simulink library "takeOffToLandingExp"  (R2020a)
settings: Solver=VariableStepAuto  StartTime=0.0  StopTime=10.0  RelTol=1e-3
undefined symbols (not defined in the file or in its folder): elSP, env, FLIGHTCONTROLLER, fltCtrl, gain2to3, gain4to1, hiLvlCtrl, initializeBussesFromBlock, pathFollowingControllerExp, pathFollowingControllerExp_cl, vhcl
libraries: simulink x9, filteredPIDController_ul x4, ctrlAllocMatrix_cl x3, velocityAngle_ul x3, hiToLoElevationControllerExp x2, takeoffToLanding_cl x2, dspsigops x1, setpointToOutput_cl x1, stopwatch_ul x1, courseFollowExp_cl x1, eulAng2RotMat_ul x1, angleBtw2Vecs_ul x1
settings Model: Creator=jcreed2  LastModifiedBy=jcreed2

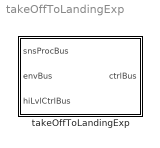
== system takeOffToLandingExp ==
  takeOffToLandingExp : Subsystem  LoadFcn=initializeBussesFromBlock(gcb)  InitFcn=initializeBussesFromBlock(gcb)  StartFcn=initializeBussesFromBlock(gcb)  mask{initPosForInitSStar=vhcl.initPosVecGnd.Value, fluidDensity=env.water.density.Value, pathCtrl=fltCtrl, aeroStruct=vhcl.struct('OCT.aeroSurf')}
      mask prompts: initPosForInitSStar "Initial Position"; fluidDensity "Fluid Density"; pathCtrl "Controller"; aeroStruct "Aerodynamic Structure"

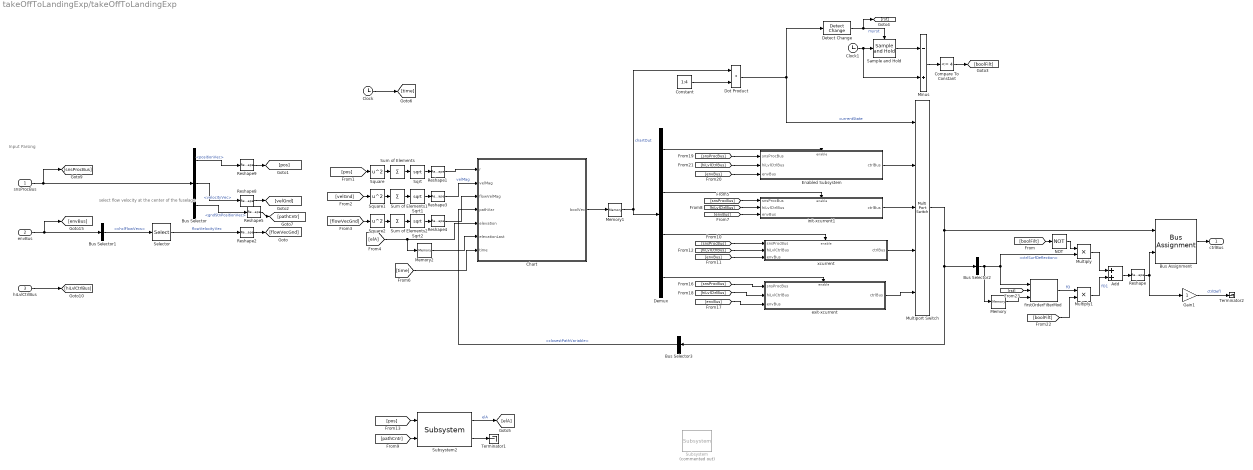
== system takeOffToLandingExp/takeOffToLandingExp ==
  note: select flow velocity at the center of the fuselage
  note: Input Parsing
  snsProcBus : Inport  OutDataTypeStr=Bus: sensorsProcessingBus
  envBus : Inport  Port=2  OutDataTypeStr=Bus: envBus
  hiLvlCtrlBus : Inport  Port=3  OutDataTypeStr=Bus: hiLvlCtrlBus
  Add : Sum
  Bus Assignment : BusAssignment  AssignedSignals=ctrlSurfDeflection
  Bus Selector : BusSelector  OutputSignals=positionVec,velocityVec,gndStnPositionVec
  Bus Selector1 : BusSelector  OutputSignals=vhclFlowVecs
  Bus Selector2 : BusSelector  OutputSignals=ctrlSurfDeflection
  Bus Selector3 : BusSelector  OutputSignals=closestPathVariable
  Chart : Stateflow chart  AncestorBlock=takeoffToLanding_cl/takeoffToLanding/Chart  TreatAsAtomicUnit=on  mask{nonCrossSpoolGain=2, gain41=gain4to1, gain23=gain2to3, maxR=3}
      mask prompts: nonCrossSpoolGain "non-xcurrent spool speed gain"; maxR "max kite position magnitude (r)"
  Clock : Clock
  Clock1 : Clock
  Compare To Constant : simulink/Logic and Bit Operations/Compare To Constant  relop=<=  const=4  OutDataTypeStr=boolean
  Constant : Constant  Value=1:4
  Demux : Demux
  Detect Change : simulink/Logic and Bit Operations/Detect Change  vinit=0  OutDataTypeStr=boolean
  Dot Product : DotProduct  InputSameDT=on  OutDataTypeStr=Inherit: Inherit via internal rule
  Enabled Subsystem : Subsystem  TreatAsAtomicUnit=on
  Gain1 : Gain
  Memory : Memory  InitialCondition=[0;0;0;0]
  Memory1 : Memory  InitialCondition=[1 0 0 0]
  Memory2 : Memory  InitialCondition=.36
  Minus : Sum  Inputs=-+
  Multiply : Product
  Multiply1 : Product
  Multiport Switch : MultiPortSwitch  Inputs=4  DataPortIndices={1,2,3,4,5,6}  DiagnosticForDefault=Warning
  NOT : Logic  Operator=NOT  AllPortsSameDT=off  OutDataTypeStr=boolean
  Reshape{,1,3..4} (4 alike) : Reshape
  Reshape{2,5,8..9} (4 alike) : Reshape  OutputDimensionality=Column vector (2-D)
  Sample and Hold : dspsigops/Sample and Hold  trig=Rising edge  initCond=0  latchinput=off
  Selector : Selector  NumberOfDimensions=2  InputPortWidth=3  IndexOptions=Select all,Index vector (dialog)  Indices=[1 3],5  OutputSizes=1,1
  Sqrt : Sqrt  SaturateOnIntegerOverflow=on
  Sqrt1 : Sqrt  SaturateOnIntegerOverflow=on
  Sqrt2 : Sqrt  SaturateOnIntegerOverflow=on
  Square : Math  Operator=square  SaturateOnIntegerOverflow=on
  Square1 : Math  Operator=square  SaturateOnIntegerOverflow=on
  Square2 : Math  Operator=square  SaturateOnIntegerOverflow=on
  Subsystem : takeoffToLanding_cl/takeoffToLanding/Subsystem  Commented=on  SystemSampleTime=-1  Latency=0  AutoFrameSizeCalculation=off
  Subsystem2 : hiToLoElevationControllerExp/hiToLoElevationControllerExp/Subsystem  SystemSampleTime=-1  Latency=0  AutoFrameSizeCalculation=off
  Sum of Elements : Sum  Inputs=+
  Sum of Elements1 : Sum  Inputs=+
  Sum of Elements2 : Sum  Inputs=+
  Terminator1 : Terminator
  Terminator2 : Terminator
  exit-xcurrent : Subsystem  AncestorBlock=takeoffToLanding_cl/takeoffToLanding/exit-xcurrent  TreatAsAtomicUnit=on
  "firstOrderFilterMod " : takeoffToLanding_cl/takeoffToLanding/firstOrderFilterMod   tau=10  ic=0
  init-xcurrent1 : Subsystem  AncestorBlock=takeoffToLanding_cl/takeoffToLanding/init-xcurrent  TreatAsAtomicUnit=on
  xcurrent : Subsystem  AncestorBlock=takeoffToLanding_cl/takeoffToLanding/xcurrent  TreatAsAtomicUnit=on
  ctrlBus : Outport  OutDataTypeStr=Bus: fltCtrlBus
  wires:
  [snsProcBus] -> exit-xcurrent/1(snsProcBus)
  [snsProcBus] -> Enabled Subsystem/1(snsProcBus)
  Reshape3/1 -> Chart/2(velMag)  "velMag"
  Multiport Switch/1 -> Bus Assignment/1, Bus Selector2/1, Bus Selector3/1
  Bus Selector2/1 -> Multiply/2, "firstOrderFilterMod "/1, Memory/1  "<ctrlSurfDeflection>"
  Multiply1/1 -> Add/2  "fO1"
  Memory1/1 -> Dot Product/1, Demux/1  "chartOut"
  Sum of Elements1/1 -> Sqrt1/1
  Clock/1 -> [time]
  Sqrt1/1 -> Reshape3/1
  [hiLvlCtrlBus] -> exit-xcurrent/2(hiLvlCtrlBus)
  [elA] -> Memory2/1, Chart/5(elevation)
  Square/1 -> Sum of Elements/1
  NOT/1 -> Multiply/1
  Reshape4/1 -> Chart/3(flowVelMag)
  Square1/1 -> Sum of Elements1/1
  Memory2/1 -> Chart/6(elevationLast)
  [time] -> Chart/7(time)
  Detect Change/1 -> [rst], Sample and Hold/Trigger  "myrst"
  Reshape/1 -> Gain1/1, Bus Assignment/2
  Square2/1 -> Sum of Elements2/1
  [velGnd] -> Square1/1
  snsProcBus/1 -> [snsProcBus], Bus Selector/1
  Multiply/1 -> Add/1
  Reshape8/1 -> [velGnd]
  hiLvlCtrlBus/1 -> [hiLvlCtrlBus]
  Bus Selector/2 -> Reshape8/1  "<velocityVec>"
  [flowVecGnd] -> Square2/1
  [boolFilt] -> NOT/1
  Sum of Elements/1 -> Sqrt/1
  Gain1/1 -> Terminator2/1  "ctrlDefl"
  Reshape1/1 -> Chart/1(r)
  [boolFilt] -> Multiply1/2
  Sqrt2/1 -> Reshape4/1
  Sqrt/1 -> Reshape1/1
  Minus/1 -> Compare To Constant/1
  Bus Selector3/1 -> Chart/4(pathVar)  "<closestPathVariable>"
  Reshape2/1 -> [flowVecGnd]
  Sum of Elements2/1 -> Sqrt2/1
  Bus Selector1/1 -> Selector/1  "<vhclFlowVecs>"
  Enabled Subsystem/1(ctrlBus) -> Multiport Switch/2
  Memory/1 -> "firstOrderFilterMod "/3
  Add/1 -> Reshape/1
  Clock1/1 -> Minus/2, Sample and Hold/1
  Compare To Constant/1 -> [boolFilt]
  [rst] -> "firstOrderFilterMod "/2
  Dot Product/1 -> Multiport Switch/1, Detect Change/1  "currentState"
  Chart/1(boolVec) -> Memory1/1
  Constant/1 -> Dot Product/2
  envBus/1 -> [envBus], Bus Selector1/1
  Sample and Hold/1 -> Minus/1
  "firstOrderFilterMod "/1 -> Multiply1/1  "fO"
  Reshape9/1 -> [pos]
  Bus Selector/1 -> Reshape9/1  "<positionVec>"
  Selector/1 -> Reshape2/1  "flowVelocityVec"
  [envBus] -> exit-xcurrent/3(envBus)
  [pos] -> Square/1
  [hiLvlCtrlBus] -> Enabled Subsystem/2(hiLvlCtrlBus)
  [envBus] -> Enabled Subsystem/3(envBus)
  [snsProcBus] -> xcurrent/1(snsProcBus)
  [hiLvlCtrlBus] -> xcurrent/2(hiLvlCtrlBus)
  [envBus] -> xcurrent/3(envBus)
  Bus Assignment/1 -> ctrlBus/1
  exit-xcurrent/1(ctrlBus) -> Multiport Switch/5
  xcurrent/1(ctrlBus) -> Multiport Switch/4
  init-xcurrent1/1(ctrlBus) -> Multiport Switch/3
  [snsProcBus] -> init-xcurrent1/1(snsProcBus)
  [hiLvlCtrlBus] -> init-xcurrent1/2(hiLvlCtrlBus)
  [envBus] -> init-xcurrent1/3(envBus)
  Demux/1 -> Enabled Subsystem/Enable
  Demux/2 -> init-xcurrent1/Enable
  Demux/3 -> xcurrent/Enable
  Demux/4 -> exit-xcurrent/Enable
  Subsystem2/1 -> [elA]  "elA"
  [pos] -> Subsystem2/1
  [pathCntr] -> Subsystem2/2
  Subsystem2/2 -> Terminator1/1
  Bus Selector/3 -> Reshape5/1  "<gndStnPositionVec>"
  Reshape5/1 -> [pathCntr]

== system takeOffToLandingExp/takeOffToLandingExp/Enabled Subsystem ==
  snsProcBus : Inport  OutDataTypeStr=Bus: sensorsProcessingBus
  hiLvlCtrlBus : Inport  Port=2  OutDataTypeStr=Bus: hiLvlCtrlBus
  envBus : Inport  Port=3  OutDataTypeStr=Bus: envBus
  Enable : EnablePort
  hiToLoElevationControllerExp : Subsystem  AncestorBlock=hiToLoElevationControllerExp/hiToLoElevationControllerExp  LoadFcn=initializeBussesFromBlock(gcb)  InitFcn=initializeBussesFromBlock(gcb)  StartFcn=initializeBussesFromBlock(gcb)  mask{initPosForInitSStar=vhcl.initPosVecGnd.Value, fluidDensity=env.water.density.Value, pathCtrl=fltCtrl, aeroStruct=vhcl.struct('OCT.aeroSurf'), thrAttach=vhcl.rBridle_LE.Value}
      mask prompts: initPosForInitSStar "Initial Position"; fluidDensity "Fluid Density"; pathCtrl "Controller"; aeroStruct "Aerodynamic Structure"; thrAttach "Tether Attach Point"
      mask DialogControl Container3 Prompt: courseFollow Params
      mask DialogControl Container4 Prompt: setpointToOutput Params
  ctrlBus : Outport  OutDataTypeStr=Bus: fltCtrlBus  VectorParamsAs1DForOutWhenUnconnected=off
  wires:
  envBus/1 -> hiToLoElevationControllerExp/3(envBus)
  hiLvlCtrlBus/1 -> hiToLoElevationControllerExp/2(hiLvlCtrlBus)
  hiToLoElevationControllerExp/1(ctrlBus) -> ctrlBus/1
  snsProcBus/1 -> hiToLoElevationControllerExp/1(snsProcBus)

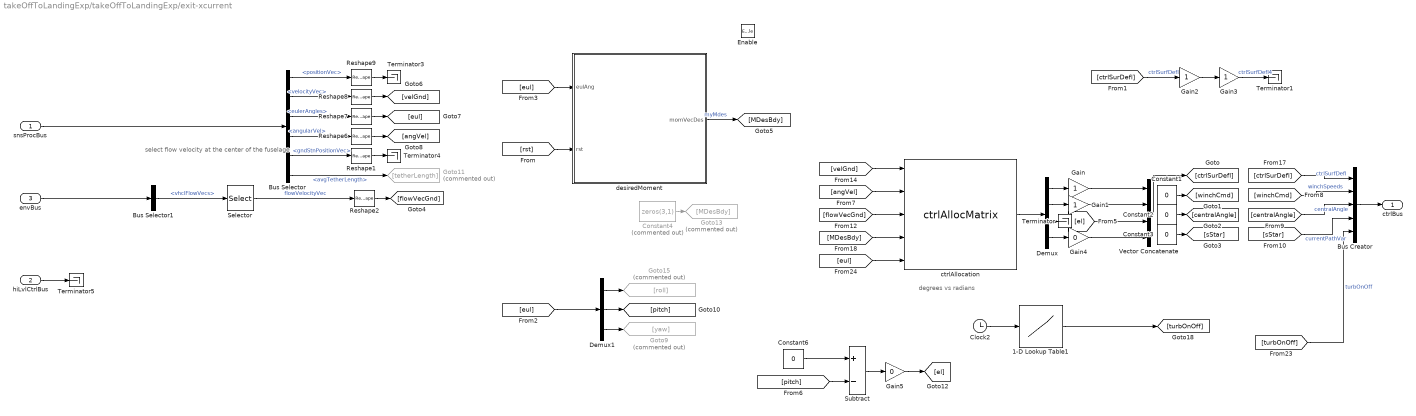
== system takeOffToLandingExp/takeOffToLandingExp/exit-xcurrent ==
  note: select flow velocity at the center of the fuselage
  note: degrees vs radians
  snsProcBus : Inport  OutDataTypeStr=Bus: sensorsProcessingBus
  hiLvlCtrlBus : Inport  Port=2  OutDataTypeStr=Bus: hiLvlCtrlBus
  envBus : Inport  Port=3  OutDataTypeStr=Bus: envBus
  Enable : EnablePort
  1-D Lookup Table1 : Lookup_n-D  NumberOfTableDimensions=1  BreakpointsForDimension1=[0 1000 2000]  Table=[0 0 0]  InterpMethod=Flat  InternalRulePriority=Speed  RndMeth=Simplest  InputSameDT=on
  Bus Creator : BusCreator  Inputs=5  OutDataTypeStr=Bus: fltCtrlBus
      settings: InheritFromInputs=off
  Bus Selector : BusSelector  OutputSignals=positionVec,velocityVec,eulerAngles,angularVel,gndStnPositionVec,avgTetherLength
  Bus Selector1 : BusSelector  OutputSignals=vhclFlowVecs
  Clock2 : Clock
  Constant{1..3,6} (4 alike) : Constant  Value=0
  Constant4 : Constant  Commented=on  Value=zeros(3,1)
  Demux : Demux
  Demux1 : Demux  Outputs=3
  Gain{,1..3} (4 alike) : Gain
  Gain4 : Gain  Gain=0
  Gain5 : Gain  Gain=0
  Goto11 : Goto  Commented=on  GotoTag=tetherLength
  Goto13 : Goto  Commented=on  GotoTag=MDesBdy
  Goto15 : Goto  Commented=on  GotoTag=roll
  Goto9 : Goto  Commented=on  GotoTag=yaw
  Reshape{1..2,6..9} (6 alike) : Reshape  OutputDimensionality=Column vector (2-D)
  Selector : Selector  NumberOfDimensions=2  InputPortWidth=3  IndexOptions=Select all,Index vector (dialog)  Indices=[1 3],5  OutputSizes=1,1
  Subtract : Sum  Inputs=+-
  Terminator{,1,3..5} (5 alike) : Terminator
  Vector Concatenate : Concatenate  NumInputs=4
  ctrlAllocation : ctrlAllocMatrix_cl/ctrlAllocMatrix  aeroStruct=aeroStruct  fluidDensity=fluidDensity
  desiredMoment : Subsystem  AncestorBlock=takeoffToLanding_cl/takeoffToLanding/non-xcurrent/desiredMoment
  ctrlBus : Outport  OutDataTypeStr=Bus: fltCtrlBus  VectorParamsAs1DForOutWhenUnconnected=off
  wires:
  Demux/3 -> Terminator/1
  [el] -> Vector Concatenate/3
  hiLvlCtrlBus/1 -> Terminator5/1
  Constant4/1 -> Goto13/1
  Demux/4 -> Gain4/1
  Demux/2 -> Gain1/1
  Demux/1 -> Gain/1
  Vector Concatenate/1 -> [ctrlSurDefl]
  ctrlAllocation/1 -> Demux/1
  Bus Selector/6 -> Goto11/1  "<avgTetherLength>"
  [velGnd] -> ctrlAllocation/1
  [MDesBdy] -> ctrlAllocation/4
  [eul] -> ctrlAllocation/5
  [angVel] -> ctrlAllocation/2
  [flowVecGnd] -> ctrlAllocation/3
  Reshape6/1 -> [angVel]
  snsProcBus/1 -> Bus Selector/1
  Reshape1/1 -> Terminator4/1
  envBus/1 -> Bus Selector1/1
  Bus Selector1/1 -> Selector/1  "<vhclFlowVecs>"
  Reshape2/1 -> [flowVecGnd]
  Bus Selector/5 -> Reshape1/1  "<gndStnPositionVec>"
  Reshape9/1 -> Terminator3/1
  Selector/1 -> Reshape2/1  "flowVelocityVec"
  Reshape8/1 -> [velGnd]
  Bus Selector/4 -> Reshape6/1  "<angularVel>"
  Reshape7/1 -> [eul]
  Bus Selector/2 -> Reshape8/1  "<velocityVec>"
  Bus Selector/3 -> Reshape7/1  "<eulerAngles>"
  Bus Selector/1 -> Reshape9/1  "<positionVec>"
  Constant3/1 -> [sStar]
  Constant2/1 -> [centralAngle]
  Constant1/1 -> [winchCmd]
  [centralAngle] -> Bus Creator/3  "centralAngle"
  Bus Creator/1 -> ctrlBus/1
  [winchCmd] -> Bus Creator/2  "winchSpeeds"
  [ctrlSurDefl] -> Bus Creator/1  "ctrlSurfDefl"
  [sStar] -> Bus Creator/4  "currentPathVar"
  Clock2/1 -> 1-D Lookup Table1/1
  [turbOnOff] -> Bus Creator/5  "turbOnOff"
  1-D Lookup Table1/1 -> [turbOnOff]
  Gain/1 -> Vector Concatenate/1
  Gain1/1 -> Vector Concatenate/2
  [rst] -> desiredMoment/2(rst)
  desiredMoment/1(momVecDes) -> [MDesBdy]  "myMdes"
  [eul] -> desiredMoment/1(eulAng)
  [ctrlSurDefl] -> Gain2/1  "ctrlSurfDefl"
  Gain2/1 -> Gain3/1
  Gain3/1 -> Terminator1/1  "ctrlSurfDefl4"
  Gain4/1 -> Vector Concatenate/4
  [eul] -> Demux1/1
  Demux1/2 -> [pitch]
  Demux1/1 -> Goto15/1
  Demux1/3 -> Goto9/1
  Constant6/1 -> Subtract/1
  [pitch] -> Subtract/2
  Gain5/1 -> [el]
  Subtract/1 -> Gain5/1

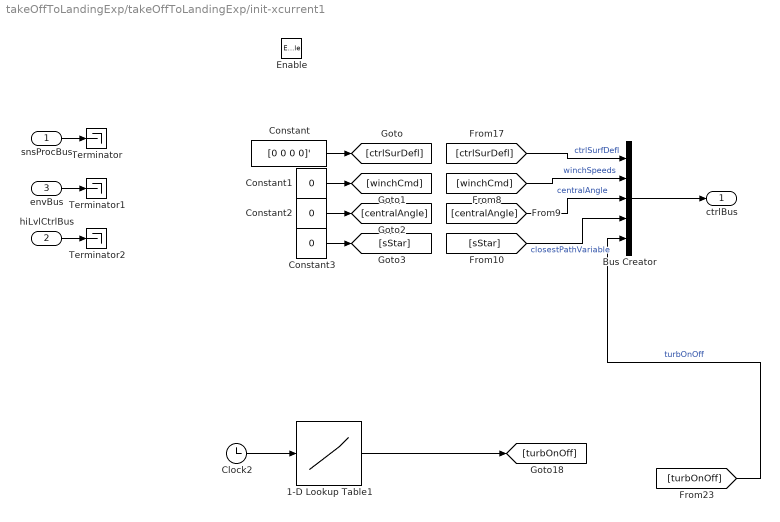
== system takeOffToLandingExp/takeOffToLandingExp/init-xcurrent1 ==
  snsProcBus : Inport  OutDataTypeStr=Bus: sensorsProcessingBus
  hiLvlCtrlBus : Inport  Port=2  OutDataTypeStr=Bus: hiLvlCtrlBus
  envBus : Inport  Port=3  OutDataTypeStr=Bus: envBus
  Enable : EnablePort
  1-D Lookup Table1 : Lookup_n-D  NumberOfTableDimensions=1  BreakpointsForDimension1=[0 1000 2000]  Table=[0 0 0]  InterpMethod=Flat  InternalRulePriority=Speed  RndMeth=Simplest  InputSameDT=on
  Bus Creator : BusCreator  Inputs=5  OutDataTypeStr=Bus: fltCtrlBus
      settings: InheritFromInputs=off
  Clock2 : Clock
  Constant : Constant  Value=[0 0 0 0]'
  Constant1 : Constant  Value=0
  Constant2 : Constant  Value=0
  Constant3 : Constant  Value=0
  Terminator : Terminator
  Terminator1 : Terminator
  Terminator2 : Terminator
  ctrlBus : Outport  OutDataTypeStr=Bus: fltCtrlBus  VectorParamsAs1DForOutWhenUnconnected=off
  wires:
  Constant/1 -> [ctrlSurDefl]
  Constant3/1 -> [sStar]
  Bus Creator/1 -> ctrlBus/1
  Constant1/1 -> [winchCmd]
  [sStar] -> Bus Creator/4  "closestPathVariable"
  snsProcBus/1 -> Terminator/1
  Constant2/1 -> [centralAngle]
  hiLvlCtrlBus/1 -> Terminator2/1
  envBus/1 -> Terminator1/1
  [winchCmd] -> Bus Creator/2  "winchSpeeds"
  [centralAngle] -> Bus Creator/3  "centralAngle"
  [ctrlSurDefl] -> Bus Creator/1  "ctrlSurfDefl"
  [turbOnOff] -> Bus Creator/5  "turbOnOff"
  Clock2/1 -> 1-D Lookup Table1/1
  1-D Lookup Table1/1 -> [turbOnOff]

== system takeOffToLandingExp/takeOffToLandingExp/xcurrent ==
  snsProcBus : Inport  OutDataTypeStr=Bus: sensorsProcessingBus
  hiLvlCtrlBus : Inport  Port=2  OutDataTypeStr=Bus: hiLvlCtrlBus
  envBus : Inport  Port=3  OutDataTypeStr=Bus: envBus
  Enable : EnablePort
  pathFollowingControllerExp : Subsystem  AncestorBlock=pathFollowingControllerExp_cl/pathFollowingControllerExp  LoadFcn=initializeBussesFromBlock(gcb)  InitFcn=initializeBussesFromBlock(gcb)  StartFcn=initializeBussesFromBlock(gcb)  VariantControl=strcmpi(FLIGHTCONTROLLER,'pathFollowingControllerMantaBandLin')  mask{initPosForInitSStar=vhcl.initPosVecGnd.Value, fluidDensity=env.water.density.Value, pathCtrl=fltCtrl, aeroStruct=vhcl.struct('OCT.aeroSurf'), thrAttach=vhcl.rBridle_LE.Value}
      mask prompts: initPosForInitSStar "Initial Position"; fluidDensity "Fluid Density"; pathCtrl "Controller"; aeroStruct "Aerodynamic Structure"; thrAttach "Tether Attach Point"
      settings: MinAlgLoopOccurrences=on
      mask DialogControl Container3 Prompt: courseFollow Params
      mask DialogControl Container4 Prompt: setpointToOutput Params
  ctrlBus : Outport  OutDataTypeStr=Bus: fltCtrlBus  VectorParamsAs1DForOutWhenUnconnected=off
  wires:
  snsProcBus/1 -> pathFollowingControllerExp/1(snsProcBus)
  hiLvlCtrlBus/1 -> pathFollowingControllerExp/2(hiLvlCtrlBus)
  envBus/1 -> pathFollowingControllerExp/3(envBus)
  pathFollowingControllerExp/1(ctrlBus) -> ctrlBus/1

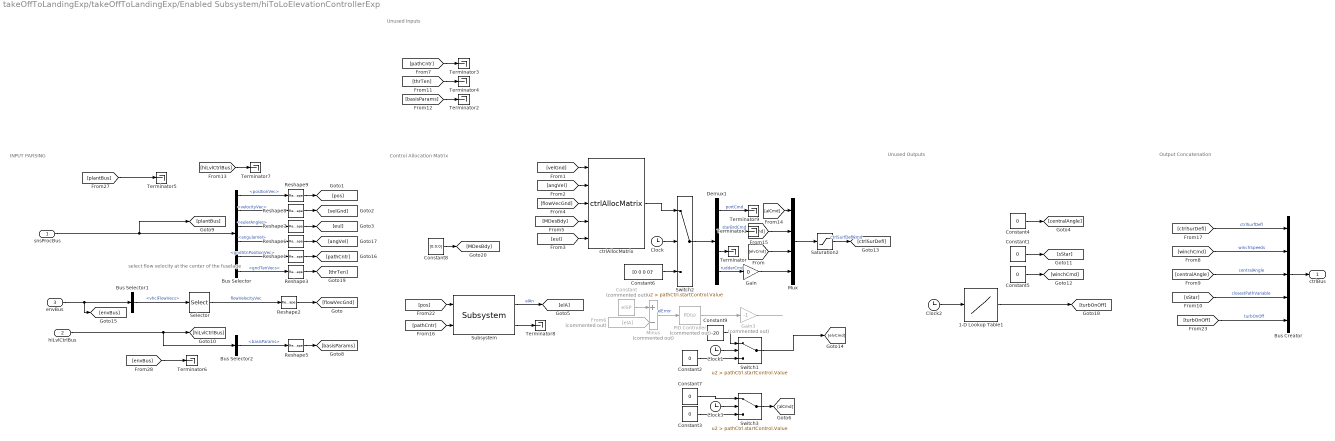
== system takeOffToLandingExp/takeOffToLandingExp/Enabled Subsystem/hiToLoElevationControllerExp ==
  note: Output Concatenation
  note: select flow velocity at the center of the fuselage
  note: INPUT PARSING
  note: Unused Outputs
  note: Control Allocation Matrix
  note: Unused Inputs
  snsProcBus : Inport  OutDataTypeStr=Bus: sensorsProcessingBus
  hiLvlCtrlBus : Inport  Port=2  OutDataTypeStr=Bus: hiLvlCtrlBus
  envBus : Inport  Port=3  OutDataTypeStr=Bus: envBus
  1-D Lookup Table1 : Lookup_n-D  NumberOfTableDimensions=1  BreakpointsForDimension1=[0 1000 2000]  Table=[0 0 0]  InterpMethod=Flat  InternalRulePriority=Speed  RndMeth=Simplest  InputSameDT=on
  Bus Creator : BusCreator  Inputs=5  OutDataTypeStr=Bus: fltCtrlBus
      settings: InheritFromInputs=off
  Bus Selector : BusSelector  OutputSignals=positionVec,velocityVec,eulerAngles,angularVel,gndStnPositionVec,gndTenVecs
  Bus Selector1 : BusSelector  OutputSignals=vhclFlowVecs
  Bus Selector2 : BusSelector  OutputSignals=basisParams
  Clock{,1..3} (4 alike) : Clock
  Constant : Constant  Commented=on  Value=elSP
  Constant{1..5,7} (6 alike) : Constant  Value=0
  Constant6 : Constant  Value=[0 0 0 0]'
  Constant8 : Constant  Value=[0;0;0]
  Constant9 : Constant  Value=-20
  Demux1 : Demux
  From6 : From  Commented=on  GotoTag=elA
  Gain : Gain  Gain=0
  Gain3 : Gain  Commented=on  Gain=-1
  Minus : Sum  Commented=on  Inputs=+-
  Mux : Mux
  PID Controller : simulink/Continuous/PID Controller  Commented=on  Controller=PD  Form=Parallel  TimeDomain=Continuous-time  UseExternalTs=off  SampleTime=-1  IntegratorMethod=Forward Euler  FilterMethod=Forward Euler  ControllerParametersSource=internal  P=1.5  I=0  D=7  UseFilter=on  N=100  TunerSelectOption=Transfer Function Based (PID Tuner App)  InitialConditionSource=internal  InitialConditionForIntegrator=0  InitialConditionForFilter=0  DifferentiatorICPrevScaledInput=0  ExternalReset=none  TrackingMode=off  Kt=1  LimitOutput=off  UpperSaturationLimit=inf  LowerSaturationLimit=-inf  LinearizeAsGain=on  AntiWindupMode=none  Kb=1  POutMin=[]  POutMax=[]  IOutMin=[]  IOutMax=[]  DOutMin=[]  DOutMax=[]  NOutMin=[]  NOutMax=[]  SumOutMin=[]  SumOutMax=[]  SaturationOutMin=[]  SaturationOutMax=[]  PParamMin=[]  PParamMax=[]  IParamMin=[]  IParamMax=[]  DParamMin=[]  DParamMax=[]  NParamMin=[]  NParamMax=[]  KbParamMin=[]  KbParamMax=[]  KtParamMin=[]  KtParamMax=[]  KbOutMin=[]  KbOutMax=[]  KtOutMin=[]  KtOutMax=[]  IntegratorOutMin=[]  IntegratorOutMax=[]  FilterOutMin=[]  FilterOutMax=[]  SumI1OutMin=[]  SumI1OutMax=[]  SumI2OutMin=[]  SumI2OutMax=[]  SumI3OutMin=[]  SumI3OutMax=[]  SumI4OutMin=[]  SumI4OutMax=[]  SumDOutMin=[]  SumDOutMax=[]  DifferentiatorOutMin=[]  DifferentiatorOutMax=[]  FilterDiffOutCoefMin=[]  FilterDiffOutCoefMax=[]  ReciprocalOutMin=[]  ReciprocalOutMax=[]  SumDenOutMin=[]  SumDenOutMax=[]  SumNumOutMin=[]  SumNumOutMax=[]  DivideOutMin=[]  DivideOutMax=[]  UdiffTsProdOutMin=[]  UdiffTsProdOutMax=[]  NTsProdOutMin=[]  NTsProdOutMax=[]  UintegralTsProdOutMin=[]  UintegralTsProdOutMax=[]  UngainTsProdOutMin=[]  UngainTsProdOutMax=[]  IntegratorContinuousStateAttributes=''  IntegratorStateMustResolveToSignalObject=off  IntegratorRTWStateStorageClass=Auto  FilterContinuousStateAttributes=''  FilterStateMustResolveToSignalObject=off  FilterRTWStateStorageClass=Auto  ParallelPVariant=InternalParameters  IdealPVariant=Disabled  IVariant=Disabled  DVariant=InternalParameters  IntegratorVariant=Disabled  SatVariant=Disabled  AWVariant=Disabled  PCopyVariant=Disabled  TRVariant=Disabled  FdbkBlocksVariant=Forward  IdealPFdbkVariant=Disabled  SatFdbkVariant=Disabled  DerivativeFilterVariant=ContFilter  NVariant=InternalParameters  NCopyVariant=Disabled  FilterICVariant=InternalICsFilter  IntegratorICVariant=Disabled  ExternalResetVariant=Disabled  TRSumVariant=Passthrough  SumFdbkVariant=Disabled  SumVariant=Sum_PD  TsampFilterVariant=InternalTs  TsampNgainVariant=Passthrough  TsampIntegralVariant=Disabled_SignalSpec
  Reshape{1..3,5..9} (8 alike) : Reshape  OutputDimensionality=Column vector (2-D)
  Saturation2 : Saturate  UpperLimit=pathCtrl.controlSigMax.upperLimit.Value  LowerLimit=pathCtrl.controlSigMax.lowerLimit.Value
  Selector : Selector  NumberOfDimensions=2  InputPortWidth=3  IndexOptions=Select all,Index vector (dialog)  Indices=[1 3],5  OutputSizes=1,1
  Subsystem : hiToLoElevationControllerExp/hiToLoElevationControllerExp/Subsystem  SystemSampleTime=-1  Latency=0  AutoFrameSizeCalculation=off
  Switch1 : Switch  Criteria=u2 > Threshold  Threshold=pathCtrl.startControl.Value
  Switch2 : Switch  Criteria=u2 > Threshold  Threshold=pathCtrl.startControl.Value
  Switch3 : Switch  Criteria=u2 > Threshold  Threshold=pathCtrl.startControl.Value
  Terminator{,1..9} (10 alike) : Terminator
  ctrlAllocMatrix : ctrlAllocMatrix_cl/ctrlAllocMatrix  aeroStruct=vhcl.struct('OCT.aeroSurf')  fluidDensity=fluidDensity
  ctrlBus : Outport  OutDataTypeStr=Bus: fltCtrlBus
  wires:
  [elvCmd] -> Mux/3
  [alCmd] -> Mux/2
  [alCmd] -> Mux/1
  Switch3/1 -> [alCmd]
  Constant7/1 -> Switch3/1
  Constant3/1 -> Switch3/3
  Clock3/1 -> Switch3/2
  Constant/1 -> Minus/1
  Minus/1 -> PID Controller/1  "elError"
  PID Controller/1 -> Gain3/1
  Gain3/1 -> ?
  Constant2/1 -> Switch1/3
  From6/1 -> Minus/2
  Clock1/1 -> Switch1/2
  [hiLvlCtrlBus] -> Terminator7/1
  envBus/1 -> Bus Selector1/1, [envBus]
  hiLvlCtrlBus/1 -> [hiLvlCtrlBus], Bus Selector2/1
  [thrTen] -> Terminator4/1
  [pathCntr] -> Terminator3/1
  [basisParams] -> Terminator2/1
  [MDesBdy] -> ctrlAllocMatrix/4
  Constant8/1 -> [MDesBdy]
  [flowVecGnd] -> ctrlAllocMatrix/3
  [eul] -> ctrlAllocMatrix/5
  [angVel] -> ctrlAllocMatrix/2
  [velGnd] -> ctrlAllocMatrix/1
  Demux1/3 -> Terminator/1
  Demux1/2 -> Terminator1/1  "starBrdCmd"
  Demux1/1 -> Terminator9/1  "portCmd"
  Gain/1 -> Mux/4
  Demux1/4 -> Gain/1  "rudderCmd"
  Mux/1 -> Saturation2/1
  Switch2/1 -> Demux1/1
  Saturation2/1 -> [ctrlSurDefl]  "ctrlSurfDeflCmd"
  Constant5/1 -> [winchCmd]
  Constant4/1 -> [centralAngle]
  Constant1/1 -> [sStar]
  Clock/1 -> Switch2/2
  Constant6/1 -> Switch2/3
  ctrlAllocMatrix/1 -> Switch2/1
  Clock2/1 -> 1-D Lookup Table1/1
  1-D Lookup Table1/1 -> [turbOnOff]
  [winchCmd] -> Bus Creator/2  "winchSpeeds"
  Bus Creator/1 -> ctrlBus/1
  [turbOnOff] -> Bus Creator/5  "turbOnOff"
  [sStar] -> Bus Creator/4  "closestPathVariable"
  [ctrlSurDefl] -> Bus Creator/1  "ctrlSurfDefl"
  [centralAngle] -> Bus Creator/3  "centralAngle"
  Reshape1/1 -> [pathCntr]
  [plantBus] -> Terminator5/1
  Bus Selector1/1 -> Selector/1  "<vhclFlowVecs>"
  [envBus] -> Terminator6/1
  Reshape5/1 -> [basisParams]
  Selector/1 -> Reshape2/1  "flowVelocityVec"
  Reshape2/1 -> [flowVecGnd]
  Bus Selector/5 -> Reshape1/1  "<gndStnPositionVec>"
  Bus Selector2/1 -> Reshape5/1  "<basisParams>"
  Bus Selector/4 -> Reshape6/1  "<angularVel>"
  Reshape7/1 -> [eul]
  Reshape6/1 -> [angVel]
  Reshape8/1 -> [velGnd]
  Reshape9/1 -> [pos]
  Bus Selector/3 -> Reshape7/1  "<eulerAngles>"
  Bus Selector/1 -> Reshape9/1  "<positionVec>"
  Bus Selector/2 -> Reshape8/1  "<velocityVec>"
  snsProcBus/1 -> Bus Selector/1, [plantBus]
  Reshape3/1 -> [thrTen]
  Bus Selector/6 -> Reshape3/1  "<gndTenVecs>"
  [pathCntr] -> Subsystem/2
  Subsystem/1 -> [elA]  "elAn"
  Subsystem/2 -> Terminator8/1
  [pos] -> Subsystem/1
  Switch1/1 -> [elvCmd]
  Constant9/1 -> Switch1/1

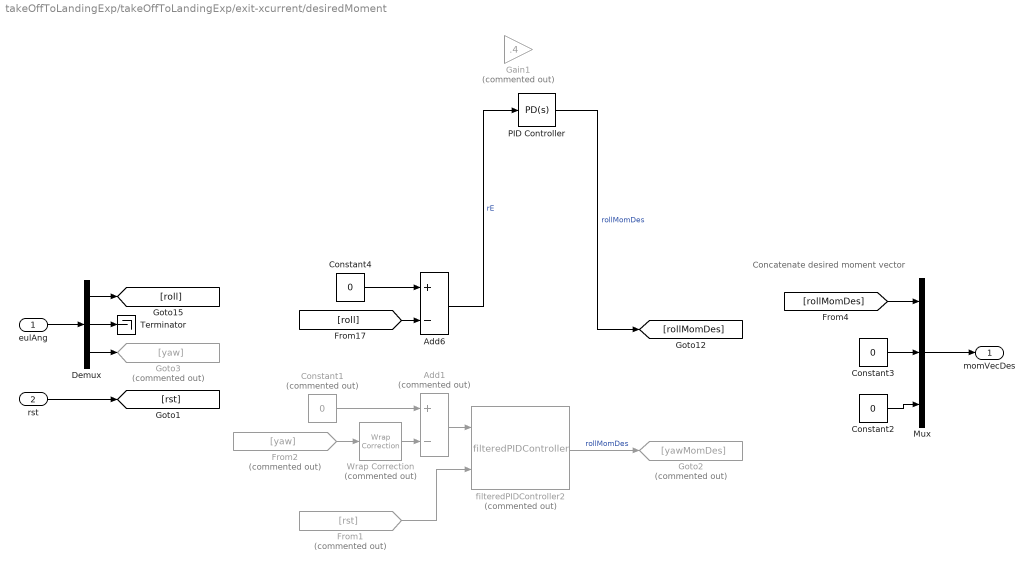
== system takeOffToLandingExp/takeOffToLandingExp/exit-xcurrent/desiredMoment ==
  note: Concatenate desired moment vector
  eulAng : Inport
  rst : Inport  Port=2
  Add1 : Sum  Commented=on  Inputs=+-
  Add6 : Sum  Inputs=+-
  Constant1 : Constant  Commented=on  Value=0
  Constant2 : Constant  Value=0
  Constant3 : Constant  Value=0
  Constant4 : Constant  Value=0
  Demux : Demux  Outputs=3
  From1 : From  Commented=on  GotoTag=rst
  From2 : From  Commented=on  GotoTag=yaw
  Gain1 : Gain  Commented=on  Gain=.4
  Goto2 : Goto  Commented=on  GotoTag=yawMomDes
  Goto3 : Goto  Commented=on  GotoTag=yaw
  Mux : Mux  Inputs=3
  PID Controller : simulink/Continuous/PID Controller  Controller=PD  Form=Parallel  TimeDomain=Continuous-time  UseExternalTs=off  SampleTime=-1  IntegratorMethod=Forward Euler  FilterMethod=Forward Euler  ControllerParametersSource=internal  P=.4  I=1  D=.1  UseFilter=on  N=100  TunerSelectOption=Transfer Function Based (PID Tuner App)  InitialConditionSource=internal  InitialConditionForIntegrator=0  InitialConditionForFilter=0  DifferentiatorICPrevScaledInput=0  ExternalReset=none  TrackingMode=off  Kt=1  LimitOutput=off  UpperSaturationLimit=inf  LowerSaturationLimit=-inf  LinearizeAsGain=on  AntiWindupMode=none  Kb=1  POutMin=[]  POutMax=[]  IOutMin=[]  IOutMax=[]  DOutMin=[]  DOutMax=[]  NOutMin=[]  NOutMax=[]  SumOutMin=[]  SumOutMax=[]  SaturationOutMin=[]  SaturationOutMax=[]  PParamMin=[]  PParamMax=[]  IParamMin=[]  IParamMax=[]  DParamMin=[]  DParamMax=[]  NParamMin=[]  NParamMax=[]  KbParamMin=[]  KbParamMax=[]  KtParamMin=[]  KtParamMax=[]  KbOutMin=[]  KbOutMax=[]  KtOutMin=[]  KtOutMax=[]  IntegratorOutMin=[]  IntegratorOutMax=[]  FilterOutMin=[]  FilterOutMax=[]  SumI1OutMin=[]  SumI1OutMax=[]  SumI2OutMin=[]  SumI2OutMax=[]  SumI3OutMin=[]  SumI3OutMax=[]  SumI4OutMin=[]  SumI4OutMax=[]  SumDOutMin=[]  SumDOutMax=[]  DifferentiatorOutMin=[]  DifferentiatorOutMax=[]  FilterDiffOutCoefMin=[]  FilterDiffOutCoefMax=[]  ReciprocalOutMin=[]  ReciprocalOutMax=[]  SumDenOutMin=[]  SumDenOutMax=[]  SumNumOutMin=[]  SumNumOutMax=[]  DivideOutMin=[]  DivideOutMax=[]  UdiffTsProdOutMin=[]  UdiffTsProdOutMax=[]  NTsProdOutMin=[]  NTsProdOutMax=[]  UintegralTsProdOutMin=[]  UintegralTsProdOutMax=[]  UngainTsProdOutMin=[]  UngainTsProdOutMax=[]  IntegratorContinuousStateAttributes=''  IntegratorStateMustResolveToSignalObject=off  IntegratorRTWStateStorageClass=Auto  FilterContinuousStateAttributes=''  FilterStateMustResolveToSignalObject=off  FilterRTWStateStorageClass=Auto  ParallelPVariant=InternalParameters  IdealPVariant=Disabled  IVariant=Disabled  DVariant=InternalParameters  IntegratorVariant=Disabled  SatVariant=Disabled  AWVariant=Disabled  PCopyVariant=Disabled  TRVariant=Disabled  FdbkBlocksVariant=Forward  IdealPFdbkVariant=Disabled  SatFdbkVariant=Disabled  DerivativeFilterVariant=ContFilter  NVariant=InternalParameters  NCopyVariant=Disabled  FilterICVariant=InternalICsFilter  IntegratorICVariant=Disabled  ExternalResetVariant=Disabled  TRSumVariant=Passthrough  SumFdbkVariant=Disabled  SumVariant=Sum_PD  TsampFilterVariant=InternalTs  TsampNgainVariant=Passthrough  TsampIntegralVariant=Disabled_SignalSpec
  Terminator : Terminator
  Wrap Correction : setpointToOutput_cl/desiredMoment/Wrap Correction  Commented=on  SystemSampleTime=-1  Latency=0  AutoFrameSizeCalculation=off
  filteredPIDController2 : filteredPIDController_ul/filteredPIDController  Commented=on  kp=pathCtrl.yawMoment.kp.Value  ki=0  kd=pathCtrl.yawMoment.kd.Value  Value=pathCtrl.yawMoment.tau.Value  externalReset=rising
  momVecDes : Outport  VectorParamsAs1DForOutWhenUnconnected=off
  wires:
  Constant2/1 -> Mux/3
  [rollMomDes] -> Mux/1
  Constant3/1 -> Mux/2
  Mux/1 -> momVecDes/1
  Demux/1 -> [roll]
  eulAng/1 -> Demux/1
  PID Controller/1 -> [rollMomDes]  "rollMomDes"
  Add6/1 -> PID Controller/1  "rE"
  [roll] -> Add6/2
  Constant4/1 -> Add6/1
  Demux/2 -> Terminator/1
  Demux/3 -> Goto3/1
  rst/1 -> [rst]
  From1/1 -> filteredPIDController2/2
  Add1/1 -> filteredPIDController2/1
  filteredPIDController2/1 -> Goto2/1  "rollMomDes"
  Constant1/1 -> Add1/1
  From2/1 -> Wrap Correction/1
  Wrap Correction/1 -> Add1/2

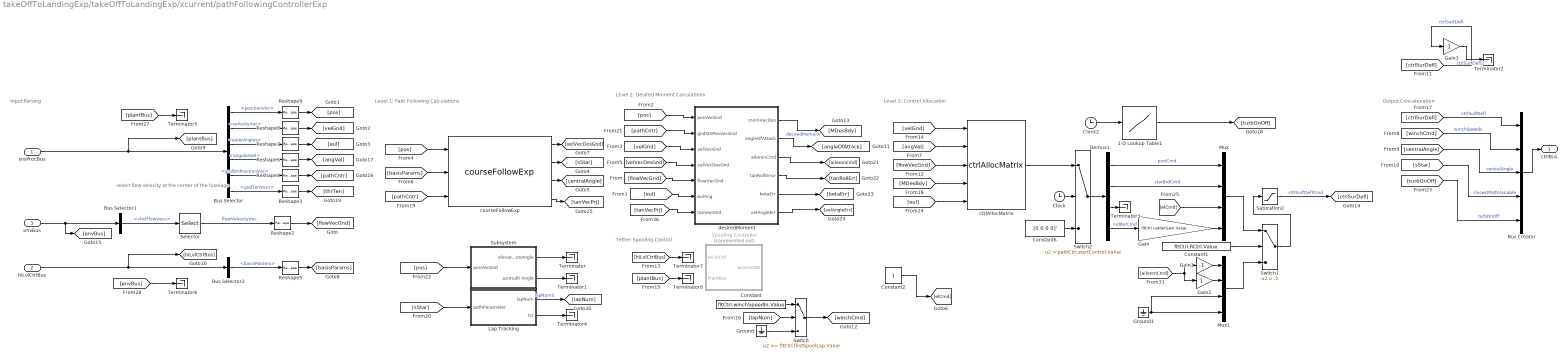
== system takeOffToLandingExp/takeOffToLandingExp/xcurrent/pathFollowingControllerExp ==
  note: Input Parsing
  note: Level 1: Path Following Calculations
  note: Level 2: Desired Moment Calculations
  note: Tether Spooling Control
  note: Output Concatenation
  note: Level 3: Control Allocation
  note: select flow velocity at the center of the fuselage
  snsProcBus : Inport  OutDataTypeStr=Bus: sensorsProcessingBus
  hiLvlCtrlBus : Inport  Port=2  OutDataTypeStr=Bus: hiLvlCtrlBus
  envBus : Inport  Port=3  OutDataTypeStr=Bus: envBus
  1-D Lookup Table1 : Lookup_n-D  NumberOfTableDimensions=1  BreakpointsForDimension1=[0 1000 2000]  Table=[0 0 0]  InterpMethod=Flat  InternalRulePriority=Speed  RndMeth=Simplest  InputSameDT=on
  Bus Creator : BusCreator  Inputs=5  OutDataTypeStr=Bus: fltCtrlBus
      settings: InheritFromInputs=off
  Bus Selector : BusSelector  OutputSignals=positionVec,velocityVec,eulerAngles,angularVel,gndStnPositionVec,gndTenVecs
  Bus Selector1 : BusSelector  OutputSignals=vhclFlowVecs
  Bus Selector2 : BusSelector  OutputSignals=basisParams
  Clock : Clock
  Clock2 : Clock
  Constant : Constant  Value=fltCtrl.winchSpeedIn.Value
  Constant1 : Constant  Value=fltCtrl.RCtrl.Value
  Constant2 : Constant
  Constant6 : Constant  Value=[0 0 0 0]'
  Demux1 : Demux
  Gain : Gain  Gain=fltCtrl.rudderGain.Value
  Gain1 : Gain  Gain=-1
  Gain2 : Gain
  Gain3 : Gain
  Ground : Ground
  Ground1 : Ground
  Lap Tracking : Subsystem
  Mux : Mux
  Mux1 : Mux
  Reshape{1..3,5..9} (8 alike) : Reshape  OutputDimensionality=Column vector (2-D)
  Saturation2 : Saturate  UpperLimit=pathCtrl.controlSigMax.upperLimit.Value  LowerLimit=pathCtrl.controlSigMax.lowerLimit.Value
  Selector : Selector  NumberOfDimensions=2  InputPortWidth=3  IndexOptions=Select all,Index vector (dialog)  Indices=[1 3],5  OutputSizes=1,1
  "Spooling Controller " : Subsystem  Commented=on
  Subsystem : Subsystem
  Switch : Switch  Threshold=fltCtrl.firstSpoolLap.Value
  Switch1 : Switch  Criteria=u2 > Threshold  Threshold=.5
  Switch2 : Switch  Criteria=u2 > Threshold  Threshold=pathCtrl.startControl.Value
  Terminator{,1..8} (9 alike) : Terminator
  courseFollowExp : courseFollowExp_cl/courseFollowExp  SystemSampleTime=-1  Latency=0  AutoFrameSizeCalculation=off
  ctrlAllocMatrix : ctrlAllocMatrix_cl/ctrlAllocMatrix  aeroStruct=vhcl.struct('OCT.aeroSurf')  fluidDensity=fluidDensity
  desiredMoment : Subsystem
  ctrlBus : Outport  OutDataTypeStr=Bus: fltCtrlBus  VectorParamsAs1DForOutWhenUnconnected=off
  wires:
  Gain3/1 -> Terminator2/1  "ctrlSurfDefl2"
  [ctrlSurDefl] -> Gain3/1  "ctrlSurfDefl"
  [tanVecPrj] -> desiredMoment/7(tanVecGnd)
  courseFollowExp/4 -> [tanVecPrj]
  desiredMoment/6(velAngleErr) -> [velAngleErr]
  desiredMoment/5(betaErr) -> [betaErr]
  desiredMoment/4(tanRollError) -> [tanRollErr]
  Switch1/1 -> Saturation2/1
  Constant1/1 -> Switch1/2
  Mux/1 -> Switch1/1
  Mux1/1 -> Switch1/3
  Ground1/1 -> Mux1/4, Mux1/3
  Gain2/1 -> Mux1/2
  Gain1/1 -> Mux1/1
  [aileronCmd] -> Gain2/1, Gain1/1
  desiredMoment/3(aileronCmd) -> [aileronCmd]
  Ground/1 -> Switch/3
  Constant/1 -> Switch/1
  [lapNum] -> Switch/2
  Switch/1 -> [winchCmd]
  [plantBus] -> Terminator8/1
  [hiLvlCtrlBus] -> Terminator7/1
  [envBus] -> Terminator6/1
  [plantBus] -> Terminator5/1
  Lap Tracking/1(lapNum) -> [lapNum]  "lapNumS"
  Lap Tracking/2(rst) -> Terminator4/1
  [sStar] -> Lap Tracking/1(pathParameter)
  Clock2/1 -> 1-D Lookup Table1/1
  1-D Lookup Table1/1 -> [turbOnOff]
  desiredMoment/2(angleOfAttack) -> [angleOfAttack]
  [elCmd] -> Mux/3
  Subsystem/2(azimuth Angle) -> Terminator1/1
  Subsystem/1(elevationAngle) -> Terminator/1
  [pos] -> Subsystem/1(posVecGnd)
  [turbOnOff] -> Bus Creator/5  "turbOnOff"
  Demux1/4 -> Gain/1  "rudderCmd"
  Gain/1 -> Mux/4
  [basisParams] -> courseFollowExp/2
  [flowVecGnd] -> desiredMoment/5(flowVecGnd)
  [eul] -> desiredMoment/6(eulAng)
  [velVecDesGnd] -> desiredMoment/4(velVecDesGnd)
  [velGnd] -> desiredMoment/3(velVecGnd)
  [pathCntr] -> desiredMoment/2(gndStnPosVecGnd)
  [pos] -> desiredMoment/1(posVecGnd)
  [pathCntr] -> courseFollowExp/3
  Bus Selector/5 -> Reshape1/1  "<gndStnPositionVec>"
  Reshape1/1 -> [pathCntr]
  Bus Selector1/1 -> Selector/1  "<vhclFlowVecs>"
  envBus/1 -> Bus Selector1/1, [envBus]
  Selector/1 -> Reshape2/1  "flowVelocityVec"
  [eul] -> ctrlAllocMatrix/5
  Reshape9/1 -> [pos]
  Reshape8/1 -> [velGnd]
  Reshape7/1 -> [eul]
  Reshape6/1 -> [angVel]
  Reshape2/1 -> [flowVecGnd]
  Saturation2/1 -> [ctrlSurDefl]  "ctrlSurfDeflCmd"
  Reshape5/1 -> [basisParams]
  Bus Selector2/1 -> Reshape5/1  "<basisParams>"
  [ctrlSurDefl] -> Bus Creator/1  "ctrlSurfDefl"
  ctrlAllocMatrix/1 -> Switch2/1
  [MDesBdy] -> ctrlAllocMatrix/4
  Constant6/1 -> Switch2/3
  Switch2/1 -> Demux1/1
  Clock/1 -> Switch2/2
  Demux1/3 -> Terminator3/1
  [flowVecGnd] -> ctrlAllocMatrix/3
  [velGnd] -> ctrlAllocMatrix/1
  [angVel] -> ctrlAllocMatrix/2
  Bus Selector/4 -> Reshape6/1  "<angularVel>"
  desiredMoment/1(momVecDes) -> [MDesBdy]  "desiredMoment"
  courseFollowExp/3 -> [centralAngle]
  [sStar] -> Bus Creator/4  "closestPathVariable"
  [centralAngle] -> Bus Creator/3  "centralAngle"
  hiLvlCtrlBus/1 -> Bus Selector2/1, [hiLvlCtrlBus]
  courseFollowExp/2 -> [sStar]
  [winchCmd] -> Bus Creator/2  "winchSpeeds"
  Bus Creator/1 -> ctrlBus/1
  [pos] -> courseFollowExp/1
  Bus Selector/3 -> Reshape7/1  "<eulerAngles>"
  Bus Selector/1 -> Reshape9/1  "<positionVec>"
  Bus Selector/2 -> Reshape8/1  "<velocityVec>"
  snsProcBus/1 -> [plantBus], Bus Selector/1
  courseFollowExp/1 -> [velVecDesGnd]
  Reshape3/1 -> [thrTen]
  Bus Selector/6 -> Reshape3/1  "<gndTenVecs>"
  Constant2/1 -> [elCmd]
  Demux1/1 -> Mux/1  "portCmd"
  Demux1/2 -> Mux/2  "starBrdCmd"

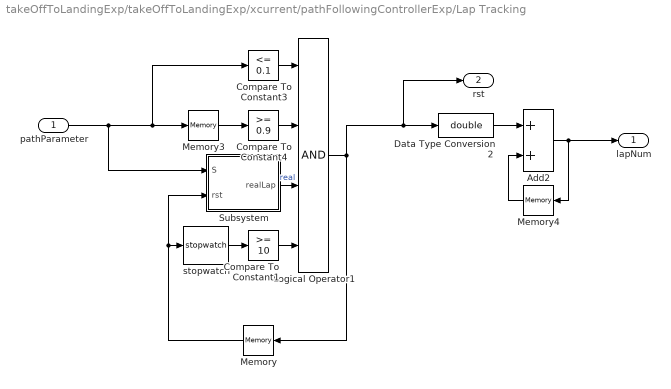
== system takeOffToLandingExp/takeOffToLandingExp/xcurrent/pathFollowingControllerExp/Lap Tracking ==
  pathParameter : Inport
  Add2 : Sum
  Compare To Constant1 : simulink/Logic and Bit Operations/Compare To Constant  relop=>=  const=10  OutDataTypeStr=boolean
  Compare To Constant3 : simulink/Logic and Bit Operations/Compare To Constant  relop=<=  const=0.1  OutDataTypeStr=boolean
  Compare To Constant4 : simulink/Logic and Bit Operations/Compare To Constant  relop=>=  const=0.9  OutDataTypeStr=boolean
  Data Type Conversion2 : DataTypeConversion  OutDataTypeStr=double
  Logical Operator1 : Logic  Inputs=4  AllPortsSameDT=off  OutDataTypeStr=boolean
  Memory : Memory  InitialCondition=false
  Memory3 : Memory
  Memory4 : Memory
  Subsystem : Subsystem
  stopwatch : stopwatch_ul/stopwatch  SystemSampleTime=-1  Latency=0  AutoFrameSizeCalculation=off
  lapNum : Outport  VectorParamsAs1DForOutWhenUnconnected=off
  rst : Outport  Port=2  VectorParamsAs1DForOutWhenUnconnected=off
  wires:
  Subsystem/1(realLap) -> Logical Operator1/3  "real"
  Compare To Constant1/1 -> Logical Operator1/4
  Memory/1 -> stopwatch/1, Subsystem/2(rst)
  stopwatch/1 -> Compare To Constant1/1
  pathParameter/1 -> Memory3/1, Compare To Constant3/1, Subsystem/1(S)
  Compare To Constant4/1 -> Logical Operator1/2
  Add2/1 -> Memory4/1, lapNum/1
  Memory4/1 -> Add2/2
  Logical Operator1/1 -> Memory/1, Data Type Conversion2/1, rst/1
  Data Type Conversion2/1 -> Add2/1
  Memory3/1 -> Compare To Constant4/1
  Compare To Constant3/1 -> Logical Operator1/1

== system takeOffToLandingExp/takeOffToLandingExp/xcurrent/pathFollowingControllerExp/Spooling Controller  ==
  HiLvlCtrl : Inport
  PlantBus : Inport  Port=2
  Add1 : Sum  Inputs=+-
  Bus Selector1 : BusSelector  OutputSignals=avgTetherLength
  Bus Selector3 : BusSelector  OutputSignals=basisParams
  Constant2 : Constant  Value=fltCtrl.optAltitude.Value
  Constant3 : Constant  Value=hiLvlCtrl.ThrCtrl.Value
  Fcn : Fcn  Expr=u(2)/sin(u(1))
  Ground : Ground
  Multiport Switch : MultiPortSwitch  DataPortOrder=Specify indices  Inputs=2  DataPortIndices={0,1}
  Mux1 : Mux  Inputs=2
  Saturation : Saturate  UpperLimit=.25  LowerLimit=-.25
  Selector2 : Selector  InputPortWidth=5  IndexOptions=Index vector (dialog)  Indices=3  OutputSizes=1
  winchCMD : Outport
  wires:
  PlantBus/1 -> Bus Selector1/1
  Constant3/1 -> Multiport Switch/1
  Saturation/1 -> Multiport Switch/2
  Ground/1 -> Multiport Switch/3
  HiLvlCtrl/1 -> Bus Selector3/1
  Multiport Switch/1 -> winchCMD/1  "winchCMD"
  Selector2/1 -> Mux1/1
  Fcn/1 -> Add1/1  "thrDes"
  Add1/1 -> Saturation/1
  Constant2/1 -> Mux1/2
  Bus Selector1/1 -> Add1/2  "<avgTetherLength>"
  Mux1/1 -> Fcn/1
  Bus Selector3/1 -> Selector2/1  "<basisParams>"

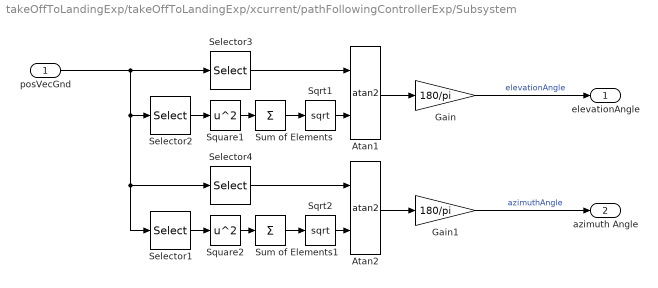
== system takeOffToLandingExp/takeOffToLandingExp/xcurrent/pathFollowingControllerExp/Subsystem ==
  posVecGnd : Inport
  Atan1 : Trigonometry  Operator=atan2
  Atan2 : Trigonometry  Operator=atan2
  Gain : Gain  Gain=180/pi
  Gain1 : Gain  Gain=180/pi
  Selector1 : Selector  InputPortWidth=3  IndexOptions=Index vector (dialog)  Indices=1  OutputSizes=1
  Selector2 : Selector  InputPortWidth=3  IndexOptions=Index vector (dialog)  Indices=[1 2]  OutputSizes=1
  Selector3 : Selector  InputPortWidth=3  IndexOptions=Index vector (dialog)  Indices=3  OutputSizes=1
  Selector4 : Selector  InputPortWidth=3  IndexOptions=Index vector (dialog)  Indices=2  OutputSizes=1
  Sqrt1 : Sqrt  SaturateOnIntegerOverflow=on
  Sqrt2 : Sqrt  SaturateOnIntegerOverflow=on
  Square1 : Math  Operator=square  SignedPower=on  SaturateOnIntegerOverflow=on
  Square2 : Math  Operator=square  SignedPower=on  SaturateOnIntegerOverflow=on
  Sum of Elements : Sum  Inputs=+
  Sum of Elements1 : Sum  Inputs=+
  elevationAngle : Outport
  azimuth Angle : Outport  Port=2
  wires:
  Gain1/1 -> azimuth Angle/1  "azimuthAngle"
  Selector4/1 -> Atan2/1
  Sqrt2/1 -> Atan2/2
  posVecGnd/1 -> Selector3/1, Selector2/1, Selector4/1, Selector1/1
  Selector1/1 -> Square2/1
  Sum of Elements1/1 -> Sqrt2/1
  Square2/1 -> Sum of Elements1/1
  Atan2/1 -> Gain1/1
  Gain/1 -> elevationAngle/1  "elevationAngle"
  Selector2/1 -> Square1/1
  Atan1/1 -> Gain/1
  Sum of Elements/1 -> Sqrt1/1
  Selector3/1 -> Atan1/1
  Square1/1 -> Sum of Elements/1
  Sqrt1/1 -> Atan1/2

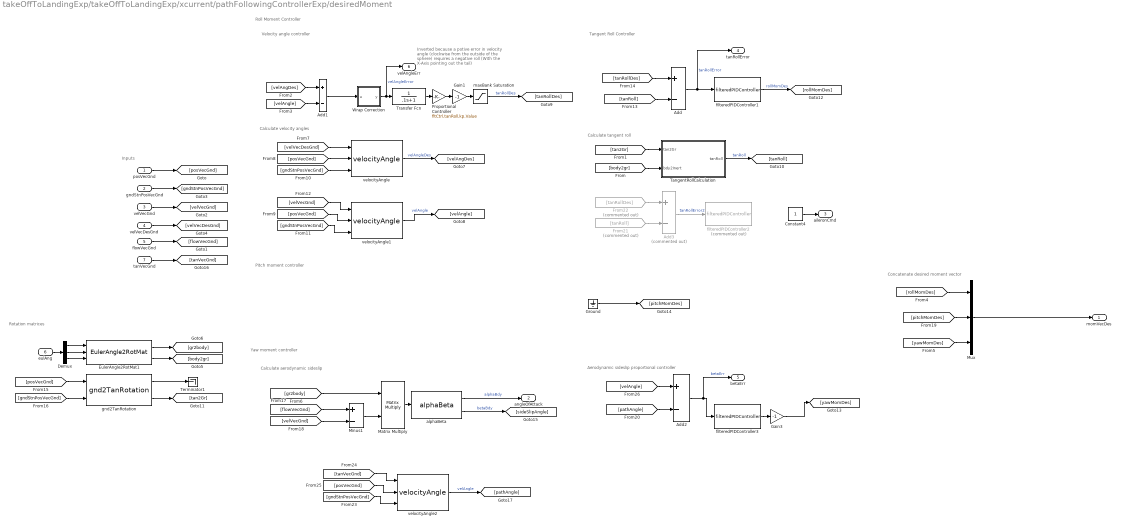
== system takeOffToLandingExp/takeOffToLandingExp/xcurrent/pathFollowingControllerExp/desiredMoment ==
  note: Calculate aerodynamic sideslip
  note: Aerodynamic sideslip proportional controller
  note: Roll Moment Controller
  note: Concatenate desired moment vector
  note: Tangent Roll Controller
  note: Calculate tangent roll
  note: Calculate velocity angles
  note: Rotation matrices
  note: Inputs
  note: Velocity angle controller
  note: Inverted because a potive error
      | in velocity angle (clockwise from the
      | outside of the sphere) requires a negative
      | roll (With the X-Axis pointing out the tail)
  note: Pitch moment controller
  note: Yaw moment controller
  posVecGnd : Inport
  gndStnPosVecGnd : Inport  Port=2
  velVecGnd : Inport  Port=3
  velVecDesGnd : Inport  Port=4
  flowVecGnd : Inport  Port=5
  eulAng : Inport  Port=6
  tanVecGnd : Inport  Port=7
  Add : Sum  Inputs=+-
  Add1 : Sum  Inputs=+-
  Add2 : Sum  Inputs=+-
  Add3 : Sum  Commented=on  Inputs=+-
  Constant4 : Constant
  Demux : Demux  Outputs=3
  EulerAngle2RotMat1 : eulAng2RotMat_ul/EulerAngle2RotMat  SystemSampleTime=-1  Latency=0  AutoFrameSizeCalculation=off
  From21 : From  Commented=on  GotoTag=tanRoll
  From22 : From  Commented=on  GotoTag=tanRollDes
  Gain1 : Gain  Gain=-1
  Gain3 : Gain  Gain=-1
  Ground : Ground
  Matrix Multiply : Product  Multiplication=Matrix(*)
  Minus1 : Sum  Inputs=+-
  Mux : Mux  Inputs=3
  Proportional Controller : Gain  Gain=fltCtrl.tanRoll.kp.Value
  TangentRollCalculation : Subsystem
  Terminator1 : Terminator
  Transfer Fcn : TransferFcn  Denominator=[.1 1]
  Wrap Correction : Subsystem
  alphaBeta : alphaBeta_ul/alphaBeta  SystemSampleTime=-1  Latency=0  AutoFrameSizeCalculation=off
  filteredPIDController1 : filteredPIDController_ul/filteredPIDController  kp=pathCtrl.rollMoment.kp.Value  ki=0  kd=pathCtrl.rollMoment.kd.Value  Value=pathCtrl.rollMoment.tau.Value  externalReset=none
  filteredPIDController2 : filteredPIDController_ul/filteredPIDController  Commented=on  kp=fltCtrl.rollCtrl.kp.Value  ki=fltCtrl.rollCtrl.ki.Value  kd=fltCtrl.rollCtrl.kd.Value  Value=fltCtrl.rollCtrl.tau.Value  externalReset=none
  filteredPIDController3 : filteredPIDController_ul/filteredPIDController  kp=pathCtrl.yawMoment.kp.Value  ki=0  kd=pathCtrl.yawMoment.kd.Value  Value=pathCtrl.yawMoment.tau.Value  externalReset=none
  gnd2TanRotation : gnd2TanRotation_ul/gnd2TanRotation  SystemSampleTime=-1  Latency=0  AutoFrameSizeCalculation=off
  maxBank Saturation : Saturate  UpperLimit=pathCtrl.maxBank.upperLimit.Value  LowerLimit=pathCtrl.maxBank.lowerLimit.Value
  velocityAngle : velocityAngle_ul/velocityAngle  SystemSampleTime=-1  Latency=0  AutoFrameSizeCalculation=off
  velocityAngle1 : velocityAngle_ul/velocityAngle  SystemSampleTime=-1  Latency=0  AutoFrameSizeCalculation=off
  velocityAngle2 : velocityAngle_ul/velocityAngle  SystemSampleTime=-1  Latency=0  AutoFrameSizeCalculation=off
  momVecDes : Outport  VectorParamsAs1DForOutWhenUnconnected=off
  angleOfAttack : Outport  Port=2  VectorParamsAs1DForOutWhenUnconnected=off
  aileronCmd : Outport  Port=3  VectorParamsAs1DForOutWhenUnconnected=off
  tanRollError : Outport  Port=4
  betaErr : Outport  Port=5
  velAngleErr : Outport  Port=6
  wires:
  filteredPIDController1/1 -> [rollMomDes]  "rollMomDes"
  Constant4/1 -> aileronCmd/1
  Gain3/1 -> [yawMomDes]
  [rollMomDes] -> Mux/1
  Mux/1 -> momVecDes/1
  Wrap Correction/1(y) -> Transfer Fcn/1, velAngleErr/1  "velAngleError"
  [posVecGnd] -> velocityAngle2/2
  [tanVecGnd] -> velocityAngle2/1
  velocityAngle2/1 -> [pathAngle]  "velAngle"
  [gndStnPosVecGnd] -> velocityAngle2/3
  tanVecGnd/1 -> [tanVecGnd]
  From22/1 -> Add3/1
  From21/1 -> Add3/2
  Add3/1 -> filteredPIDController2/1  "tanRollError2"
  Transfer Fcn/1 -> Proportional Controller/1
  Ground/1 -> [pitchMomDes]
  posVecGnd/1 -> [posVecGnd]
  velVecGnd/1 -> [velVecGnd]
  Add/1 -> filteredPIDController1/1, tanRollError/1  "tanRollError"
  Proportional Controller/1 -> Gain1/1
  Gain1/1 -> maxBank Saturation/1
  maxBank Saturation/1 -> [tanRollDes]  "tanRollDes"
  Add1/1 -> Wrap Correction/1(u)
  flowVecGnd/1 -> [flowVecGnd]
  [tan2Gr] -> TangentRollCalculation/1(tan2Gr)
  TangentRollCalculation/1(tanRoll) -> [tanRoll]  "tanRoll"
  filteredPIDController3/1 -> Gain3/1
  Minus1/1 -> Matrix Multiply/2
  [velVecGnd] -> Minus1/2
  [flowVecGnd] -> Minus1/1
  eulAng/1 -> Demux/1
  Demux/3 -> EulerAngle2RotMat1/3
  Demux/1 -> EulerAngle2RotMat1/1
  Demux/2 -> EulerAngle2RotMat1/2
  EulerAngle2RotMat1/2 -> [body2gr]
  EulerAngle2RotMat1/1 -> [gr2body]
  [body2gr] -> TangentRollCalculation/2(bdy2Inert)
  [gr2body] -> Matrix Multiply/1
  Matrix Multiply/1 -> alphaBeta/1
  alphaBeta/2 -> [sideSlipAngle]  "betaBdy"
  Add2/1 -> filteredPIDController3/1, betaErr/1  "betaErr"
  [velAngle] -> Add2/1
  alphaBeta/1 -> angleOfAttack/1  "alphaBdy"
  [pitchMomDes] -> Mux/2
  gndStnPosVecGnd/1 -> [gndStnPosVecGnd]
  velVecDesGnd/1 -> [velVecDesGnd]
  velocityAngle/1 -> [velAngDes]  "velAngleDes"
  velocityAngle1/1 -> [velAngle]  "velAngle"
  [velAngDes] -> Add1/1
  [velAngle] -> Add1/2
  [velVecDesGnd] -> velocityAngle/1
  [posVecGnd] -> velocityAngle/2
  [posVecGnd] -> velocityAngle1/2
  [gndStnPosVecGnd] -> velocityAngle/3
  [gndStnPosVecGnd] -> velocityAngle1/3
  [velVecGnd] -> velocityAngle1/1
  [tanRoll] -> Add/2
  [tanRollDes] -> Add/1
  [posVecGnd] -> gnd2TanRotation/1
  [gndStnPosVecGnd] -> gnd2TanRotation/2
  gnd2TanRotation/2 -> [tan2Gr]
  gnd2TanRotation/1 -> Terminator1/1
  [yawMomDes] -> Mux/3
  [pathAngle] -> Add2/2

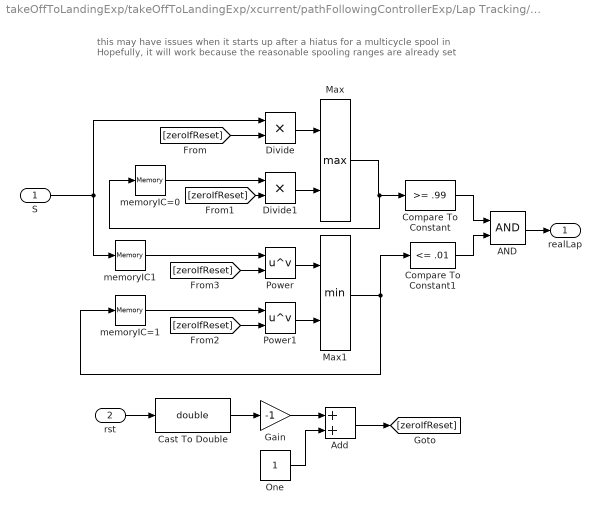
== system takeOffToLandingExp/takeOffToLandingExp/xcurrent/pathFollowingControllerExp/Lap Tracking/Subsystem ==
  note: this may have issues when it starts up after a hiatus for a multicycle spool in
      | Hopefully, it will work because the reasonable spooling ranges are already set
  S : Inport
  rst : Inport  Port=2
  AND : Logic  AllPortsSameDT=off  OutDataTypeStr=boolean
  Add : Sum
  Cast To Double : DataTypeConversion  OutDataTypeStr=double
  Compare To Constant : simulink/Logic and Bit Operations/Compare To Constant  relop=>=  const=.99  OutDataTypeStr=boolean
  Compare To Constant1 : simulink/Logic and Bit Operations/Compare To Constant  relop=<=  const=.01  OutDataTypeStr=boolean
  Divide : Product  Inputs=**
  Divide1 : Product  Inputs=**
  Gain : Gain  Gain=-1
  Max : MinMax  Function=max  Inputs=2
  Max1 : MinMax  Inputs=2
  One : Constant  OutDataTypeStr=Inherit: Inherit via back propagation
  Power : Math  Operator=pow  SaturateOnIntegerOverflow=on
  Power1 : Math  Operator=pow  SaturateOnIntegerOverflow=on
  memoryIC1 : Memory  InitialCondition=1
  memoryIC=0 : Memory
  memoryIC=1 : Memory  InitialCondition=1
  realLap : Outport
  wires:
  memoryIC1/1 -> Power/1
  memoryIC=1/1 -> Power1/1
  [zeroIfReset] -> Power1/2
  memoryIC=0/1 -> Divide1/1
  Divide1/1 -> Max/2
  [zeroIfReset] -> Divide1/2
  [zeroIfReset] -> Power/2
  [zeroIfReset] -> Divide/2
  AND/1 -> realLap/1
  Compare To Constant1/1 -> AND/2
  Compare To Constant/1 -> AND/1
  Cast To Double/1 -> Gain/1
  Power1/1 -> Max1/2
  Power/1 -> Max1/1
  Max/1 -> Compare To Constant/1, memoryIC=0/1
  Divide/1 -> Max/1
  One/1 -> Add/2
  Add/1 -> [zeroIfReset]
  Gain/1 -> Add/1
  S/1 -> memoryIC1/1, Divide/1
  rst/1 -> Cast To Double/1
  Max1/1 -> memoryIC=1/1, Compare To Constant1/1

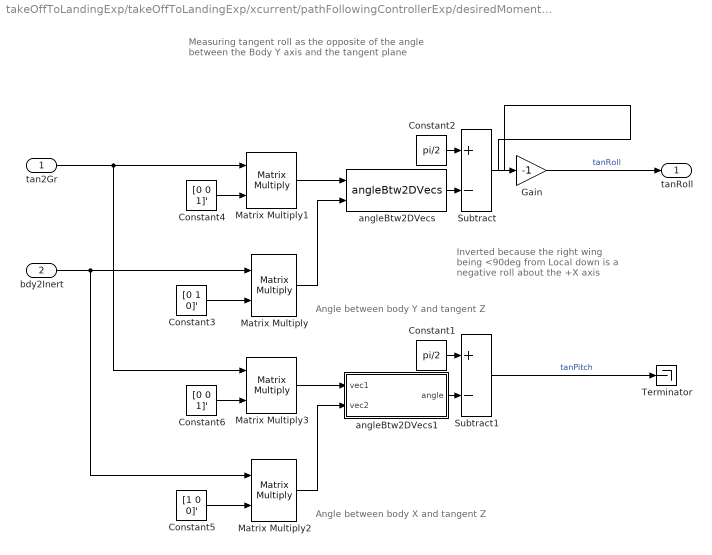
== system takeOffToLandingExp/takeOffToLandingExp/xcurrent/pathFollowingControllerExp/desiredMoment/TangentRollCalculation ==
  note: Measuring tangent roll as the opposite
      | of the angle between the Body Y axis
      | and the tangent plane
  note: Angle between body Y and tangent Z
  note: Inverted because the right wing
      | being <90deg from Local down
      | is a negative roll about the +X axis
  note: Angle between body X and tangent Z
  tan2Gr : Inport
  bdy2Inert : Inport  Port=2
  Constant1 : Constant  Value=pi/2
  Constant2 : Constant  Value=pi/2
  Constant3 : Constant  Value=[0 1 0]'
  Constant4 : Constant  Value=[0 0 1]'
  Constant5 : Constant  Value=[1 0 0]'
  Constant6 : Constant  Value=[0 0 1]'
  Gain : Gain  Gain=-1
  Matrix Multiply{,1..3} (4 alike) : Product  Multiplication=Matrix(*)
  Subtract : Sum  Inputs=+-
  Subtract1 : Sum  Inputs=+-
  Terminator : Terminator
  angleBtw2DVecs : angleBtw2Vecs_ul/angleBtw2DVecs  SystemSampleTime=-1  Latency=0  AutoFrameSizeCalculation=off
  angleBtw2DVecs1 : Subsystem
  tanRoll : Outport  VectorParamsAs1DForOutWhenUnconnected=off
  wires:
  Subtract/1 -> Gain/1
  Constant3/1 -> Matrix Multiply/2
  angleBtw2DVecs/1 -> Subtract/2
  Constant2/1 -> Subtract/1
  Matrix Multiply1/1 -> angleBtw2DVecs/1
  Constant4/1 -> Matrix Multiply1/2
  Matrix Multiply/1 -> angleBtw2DVecs/2
  Gain/1 -> tanRoll/1  "tanRoll"
  bdy2Inert/1 -> Matrix Multiply2/1, Matrix Multiply/1
  Subtract1/1 -> Terminator/1  "tanPitch"
  tan2Gr/1 -> Matrix Multiply3/1, Matrix Multiply1/1
  Matrix Multiply2/1 -> angleBtw2DVecs1/2(vec2)
  Constant6/1 -> Matrix Multiply3/2
  Matrix Multiply3/1 -> angleBtw2DVecs1/1(vec1)
  Constant1/1 -> Subtract1/1
  angleBtw2DVecs1/1(angle) -> Subtract1/2
  Constant5/1 -> Matrix Multiply2/2

== system takeOffToLandingExp/takeOffToLandingExp/xcurrent/pathFollowingControllerExp/desiredMoment/Wrap Correction ==
  note: output = mod(input-pi,2*pi)-pi
      | wraps output to -pi to pi
      |
      | ex) 1.5*pi will become -.5pi
      | 	and -1.5pi will become .5pi
      |
      | to visualize, plot the fuction above
  u : Inport
  Add1 : Sum  Inputs=+-
  Add2 : Sum  Inputs=+-
  Constant1 : Constant  Value=pi
  Constant2 : Constant  Value=2*pi
  Constant3 : Constant  Value=pi
  Mod : Math  Operator=mod  SignedPower=on  SaturateOnIntegerOverflow=on
  y : Outport  VectorParamsAs1DForOutWhenUnconnected=off
  wires:
  u/1 -> Add1/1
  Constant1/1 -> Add1/2
  Add1/1 -> Mod/1
  Constant2/1 -> Mod/2
  Mod/1 -> Add2/1  "always_pos"
  Constant3/1 -> Add2/2
  Add2/1 -> y/1

== system takeOffToLandingExp/takeOffToLandingExp/xcurrent/pathFollowingControllerExp/desiredMoment/TangentRollCalculation/angleBtw2DVecs1 ==
  vec1 : Inport
  vec2 : Inport  Port=2
  Abs : Abs
  Atan2 : Trigonometry  Operator=atan2
  Cross Product : vrlib/Utilities/Cross Product
      settings: SourceProductBaseCode=VR
  Dot Product : DotProduct  InputSameDT=on  OutDataTypeStr=Inherit: Inherit via internal rule
  Dot Product1 : DotProduct  InputSameDT=on  OutDataTypeStr=Inherit: Inherit via internal rule
  Sqrt : Sqrt  SaturateOnIntegerOverflow=on
  angle : Outport  VectorParamsAs1DForOutWhenUnconnected=off
  wires:
  Atan2/1 -> Abs/1
  vec1/1 -> Dot Product/1, Cross Product/2
  vec2/1 -> Cross Product/1, Dot Product/2
  Cross Product/1 -> Dot Product1/1, Dot Product1/2
  Dot Product/1 -> Atan2/2
  Abs/1 -> angle/1
  Dot Product1/1 -> Sqrt/1
  Sqrt/1 -> Atan2/1

== stateflow chart takeOffToLandingExp/Chart ==
  state initCC
    boolVec=[0 1 0 0];
  state crossC
    boolVec=[0 0 1 0];
  state hiToLo
    boolVec=[1 0  0 0];
  state exitC
    boolVec=[0 0 0 1];
  (default) -> hiToLo
  hiToLo -> initCC : [and(time<250,elevation>-20)]
  initCC -> crossC : [velMag>flowVelMag*.25]
  crossC -> exitC : [and(time>270,or( and(pathVar< .3,pathVar<.4),and(pathVar > .8,pathVar<.9)) )]
  data: boolVec output; r input; velMag input; flowVelMag input; nonCrossSpoolGain parameter; maxR parameter; pathVar input; elevation input; elevationLast input; time input; gain41 parameter; gain23 parameter
